simulink model "bh_test_J_DBL_pend"  (R2016b)
settings: Solver=ode15s  StartTime=0.0  StopTime=30  MaxStep=0.01  RelTol=1e-5  EnableMultiTasking=on
undefined symbols (not defined in the file or in its folder): g, L1x, L1y, L1z, L2x, L2y, L2z, mass1, mass2, theta1_0, theta2_0, X, Y, Z
undefined symbols (not defined in the file): dt
libraries: nesl_utility x14, sm_lib x12, simulink_extras x4, simulink x2
settings Model: Creator=bhorton  LastModifiedBy=bhorton
settings OptimizationCC: LifeSpan=inf
settings DebuggingCC: SFUnexpectedBacktrackingDiag=warning  SFNoUnconditionalDefaultTransitionDiag=warning  SFExecutionAtInitializationDiag=none
settings GRTTargetCC: TargetLangStandard=C89/C90 (ANSI)  GeneratePreprocessorConditionals=Disable all
settings ConfigComp: CovMetricSettings=dw  CovHtmlReporting=on  CovSaveCumulativeToWorkspaceVar=on  CovSaveSingleToWorkspaceVar=on  CovExternalEMLEnable=off

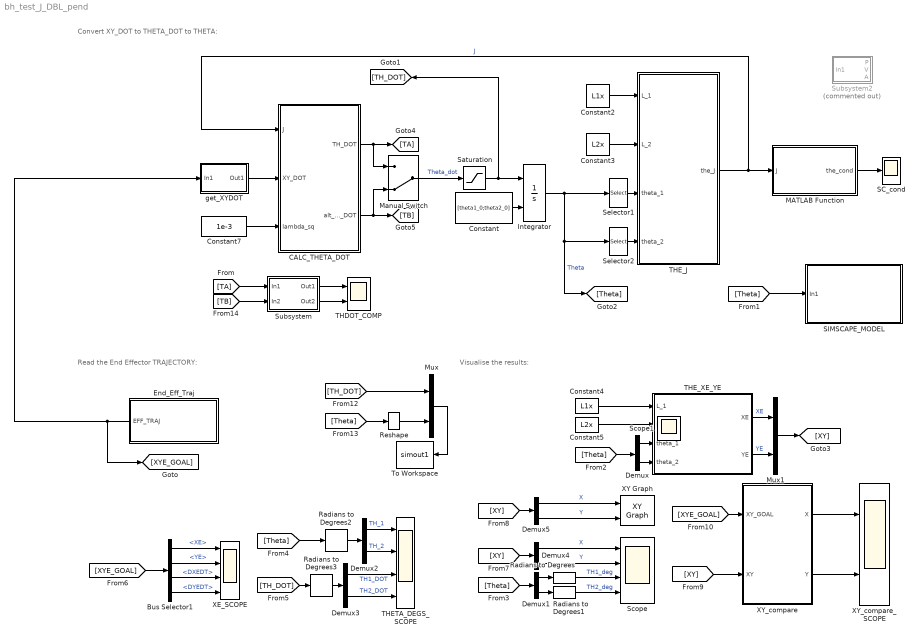
== system bh_test_J_DBL_pend ==
  note: Visualise the results:
  note: Read the End Effector TRAJECTORY:
  note: Convert XY_DOT to THETA_DOT to THETA:
  Bus Selector1 : BusSelector  OutputSignals=XE,YE,DXEDT,DYEDT
  CALC_THETA_DOT : MATLAB Function  TreatAsAtomicUnit=on
  Constant : Constant  Value=[theta1_0;theta2_0]  VectorParams1D=off
  Constant2 : Constant  Value=L1x
  Constant3 : Constant  Value=L2x
  Constant4 : Constant  Value=L1x
  Constant5 : Constant  Value=L2x
  Constant7 : Constant  Value=1e-3
  Demux{,1..5} (6 alike) : Demux  Outputs=2
  End_Eff_Traj : Subsystem
  Integrator : Integrator  InitialConditionSource=external
  MATLAB Function : MATLAB Function  TreatAsAtomicUnit=on
  Manual Switch : ManualSwitch  CurrentSetting=0
  Mux : Mux  Inputs=2
  Mux1 : Mux  Inputs=2
  Radians to Degrees{,1..3} (4 alike) : simulink_extras/Transformations/Radians to Degrees
  Reshape : Reshape
  SC_cond : Scope
  SIMSCAPE_MODEL : Subsystem
  Saturation : Saturate  UpperLimit=6  LowerLimit=-6
  Scope : Scope  NumInputPorts=4
  Selector1 : Selector  InputPortWidth=2  IndexOptions=Index vector (dialog)  Indices=1  OutputSizes=1
  Selector2 : Selector  InputPortWidth=2  IndexOptions=Index vector (dialog)  Indices=2  OutputSizes=1
  Subsystem : Subsystem
  Subsystem2 : Subsystem  Commented=on
  THDOT_COMP : Scope  NumInputPorts=2
  THETA_DEGS_SCOPE : Scope  NumInputPorts=4
  THE_J : MATLAB Function  TreatAsAtomicUnit=on
  THE_XE_YE : MATLAB Function  TreatAsAtomicUnit=on
  To Workspace : ToWorkspace  VariableName=simout1  SaveFormat=Structure With Time  SampleTime=-1
      settings: Save2DSignal=2-D array (concatenate along first dimension)
  XE_SCOPE : Scope  NumInputPorts=4
  XY Graph : simulink/Sinks/XY Graph  xmin=0  xmax=1.6  ymin=0  ymax=1.6  st=-1
  XY_compare : Subsystem
  XY_compare_SCOPE : Scope  NumInputPorts=2
  get_XYDOT : Subsystem
  Scope1 : Scope
  wires:
  Constant/1 -> Integrator/2
  Constant3/1 -> THE_J/2(L_2)
  Constant2/1 -> THE_J/1(L_1)
  THE_J/1(the_J) -> CALC_THETA_DOT/1(J), MATLAB Function/1(J)  "J"
  get_XYDOT/1(Out1) -> CALC_THETA_DOT/2(XY_DOT)
  Manual Switch/1 -> Saturation/1  "Theta_dot"
  Constant5/1 -> THE_XE_YE/2(L_2)
  Constant4/1 -> THE_XE_YE/1(L_1)
  MATLAB Function/1(the_cond) -> SC_cond/1
  Integrator/1 -> Selector2/1, [Theta], Selector1/1  "Theta"
  Selector1/1 -> THE_J/3(theta_1)
  Selector2/1 -> THE_J/4(theta_2)
  Demux/1 -> THE_XE_YE/3(theta_1)
  Demux/2 -> THE_XE_YE/4(theta_2)
  [Theta] -> Demux/1
  [Theta] -> Demux1/1
  Demux1/1 -> Radians to Degrees/1
  Demux1/2 -> Radians to Degrees1/1
  [Theta] -> SIMSCAPE_MODEL/1(In1)
  Demux2/1 -> THETA_DEGS_SCOPE/1  "TH_1"
  Demux2/2 -> THETA_DEGS_SCOPE/2  "TH_2"
  [Theta] -> Radians to Degrees2/1
  Demux3/1 -> THETA_DEGS_SCOPE/3  "TH1_DOT"
  Demux3/2 -> THETA_DEGS_SCOPE/4  "TH2_DOT"
  [TH_DOT] -> Radians to Degrees3/1
  Radians to Degrees2/1 -> Demux2/1
  Radians to Degrees3/1 -> Demux3/1
  [XYE_GOAL] -> Bus Selector1/1
  Bus Selector1/1 -> XE_SCOPE/1  "<XE>"
  Bus Selector1/2 -> XE_SCOPE/2  "<YE>"
  Bus Selector1/3 -> XE_SCOPE/3  "<DXEDT>"
  Bus Selector1/4 -> XE_SCOPE/4  "<DYEDT>"
  THE_XE_YE/1(XE) -> Mux1/1  "XE"
  THE_XE_YE/2(YE) -> Mux1/2  "YE"
  Mux1/1 -> [XY]
  Radians to Degrees1/1 -> Scope/4  "TH2_deg"
  Radians to Degrees/1 -> Scope/3  "TH1_deg"
  [XY] -> Demux4/1
  Demux4/1 -> Scope/1  "X"
  Demux4/2 -> Scope/2  "Y"
  [XY] -> Demux5/1
  Demux5/1 -> XY Graph/1  "X"
  Demux5/2 -> XY Graph/2  "Y"
  [XY] -> XY_compare/2(XY)
  [XYE_GOAL] -> XY_compare/1(XY_GOAL)
  XY_compare/2(Y) -> XY_compare_SCOPE/2
  XY_compare/1(X) -> XY_compare_SCOPE/1
  End_Eff_Traj/1(EFF_TRAJ) -> [XYE_GOAL], get_XYDOT/1(In1)
  Saturation/1 -> [TH_DOT], Integrator/1
  [TH_DOT] -> Mux/1
  Mux/1 -> To Workspace/1
  [Theta] -> Reshape/1
  Reshape/1 -> Mux/2
  [TB] -> Subsystem/2(In2)
  [TA] -> Subsystem/1(In1)
  Subsystem/1(Out1) -> THDOT_COMP/1
  Subsystem/2(Out2) -> THDOT_COMP/2
  CALC_THETA_DOT/1(TH_DOT) -> [TA], Manual Switch/1
  CALC_THETA_DOT/2(alt_TH_DOT) -> [TB], Manual Switch/2
  Constant7/1 -> CALC_THETA_DOT/3(lambda_sq)

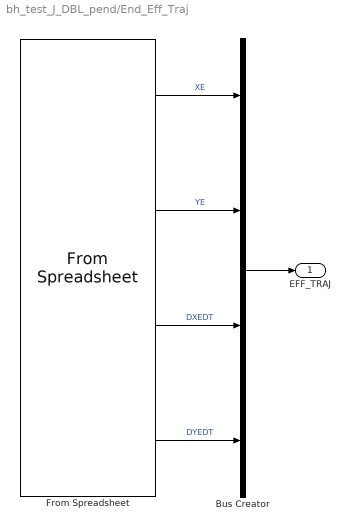
== system bh_test_J_DBL_pend/End_Eff_Traj ==
  Bus Creator : BusCreator  Inputs=4
  From Spreadsheet : FromSpreadsheet  FileName=bh_hello_complete.xlsx  SheetName=COMP_SPLINE  SampleTime=-1  ExtrapolationBeforeFirstDataPoint=Hold first value  ExtrapolationAfterLastDataPoint=Hold last value
  EFF_TRAJ : Outport
  wires:
  From Spreadsheet/2 -> Bus Creator/2  "YE"
  From Spreadsheet/3 -> Bus Creator/3  "DXEDT"
  From Spreadsheet/1 -> Bus Creator/1  "XE"
  From Spreadsheet/4 -> Bus Creator/4  "DYEDT"
  Bus Creator/1 -> EFF_TRAJ/1

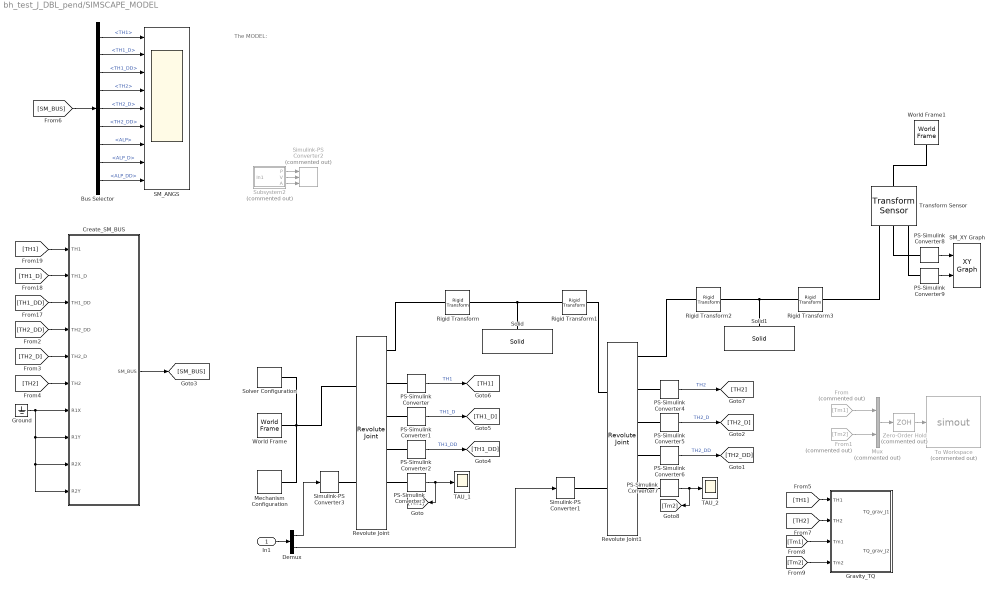
== system bh_test_J_DBL_pend/SIMSCAPE_MODEL ==
  note: The MODEL:
  In1 : Inport
  Bus Selector : BusSelector  OutputSignals=TH1,TH1_D,TH1_DD,TH2,TH2_D,TH2_DD,ALP,ALP_D,ALP_DD
  Create_SM_BUS : Subsystem
  Demux : Demux  Outputs=2
  From : From  Commented=on  GotoTag=Tm1
  From1 : From  Commented=on  GotoTag=Tm2
  Gravity_TQ : Subsystem
  Ground : Ground
  Mechanism Configuration : sm_lib/Utilities/Mechanism Configuration  UniformGravity=Constant  GravityVector=[0 -9.80665 0 ]  GravityUnits=m/s^2  LinearizationDelta=0.001
  Mux : Mux  Commented=on  Inputs=2
  PS-Simulink Converter : nesl_utility/PS-Simulink Converter  PhysicalDomain=network_engine_domain  SubClassName=ps_output  LeftPortType=input  RightPortType=output  PseudoPeriodic=off  Frequencies=[]  Unit=rad  AffineConversion=off
  PS-Simulink Converter1 : nesl_utility/PS-Simulink Converter  PhysicalDomain=network_engine_domain  SubClassName=ps_output  LeftPortType=input  RightPortType=output  PseudoPeriodic=off  Frequencies=[]  Unit=rad/s  AffineConversion=off
  PS-Simulink Converter2 : nesl_utility/PS-Simulink Converter  PhysicalDomain=network_engine_domain  SubClassName=ps_output  LeftPortType=input  RightPortType=output  PseudoPeriodic=off  Frequencies=[]  Unit=rad/s^2  AffineConversion=off
  PS-Simulink Converter3 : nesl_utility/PS-Simulink Converter  PhysicalDomain=network_engine_domain  SubClassName=ps_output  LeftPortType=input  RightPortType=output  PseudoPeriodic=off  Frequencies=[]  Unit=N*m  AffineConversion=off
  PS-Simulink Converter4 : nesl_utility/PS-Simulink Converter  PhysicalDomain=network_engine_domain  SubClassName=ps_output  LeftPortType=input  RightPortType=output  PseudoPeriodic=off  Frequencies=[]  Unit=rad  AffineConversion=off
  PS-Simulink Converter5 : nesl_utility/PS-Simulink Converter  PhysicalDomain=network_engine_domain  SubClassName=ps_output  LeftPortType=input  RightPortType=output  PseudoPeriodic=off  Frequencies=[]  Unit=rad/s  AffineConversion=off
  PS-Simulink Converter6 : nesl_utility/PS-Simulink Converter  PhysicalDomain=network_engine_domain  SubClassName=ps_output  LeftPortType=input  RightPortType=output  PseudoPeriodic=off  Frequencies=[]  Unit=rad/s^2  AffineConversion=off
  PS-Simulink Converter7 : nesl_utility/PS-Simulink Converter  PhysicalDomain=network_engine_domain  SubClassName=ps_output  LeftPortType=input  RightPortType=output  PseudoPeriodic=off  Frequencies=[]  Unit=N*m  AffineConversion=off
  PS-Simulink Converter8 : nesl_utility/PS-Simulink Converter  PhysicalDomain=network_engine_domain  SubClassName=ps_output  LeftPortType=input  RightPortType=output  PseudoPeriodic=off  Frequencies=[]  Unit=m  AffineConversion=off
  PS-Simulink Converter9 : nesl_utility/PS-Simulink Converter  PhysicalDomain=network_engine_domain  SubClassName=ps_output  LeftPortType=input  RightPortType=output  PseudoPeriodic=off  Frequencies=[]  Unit=m  AffineConversion=off
  Revolute Joint : sm_lib/Joints/Revolute Joint  SenseConstraintForce=on  SenseConstraintForceX=off  SenseConstraintForceY=off  SenseConstraintForceZ=off  SenseConstraintTorque=off  SenseConstraintTorqueX=off  SenseConstraintTorqueY=off  SenseConstraintTorqueZ=off  SenseTotalForce=off  SenseTotalForceX=off  SenseTotalForceY=off  SenseTotalForceZ=off  SenseTotalTorque=off  SenseTotalTorqueX=off  SenseTotalTorqueY=off  SenseTotalTorqueZ=off  CompositeWrenchDir=BaseOnFollower  CompositeWrenchFrame=BaseFrame  EquilibriumPosition=0  EquilibriumPositionUnits=deg  SpringStiffness=0  SpringStiffnessUnits=N*m/deg  DampingCoefficient=b1_damp  DampingCoefficientUnits=N*m/(rad/s)  TorqueActuationMode=ComputedTorque  MotionActuationMode=InputMotion  SensePosition=on  SenseVelocity=on  SenseAcceleration=on  SenseTorqueForce=on  PositionTargetSpecify=off  PositionTargetPriority=Low  PositionTargetValue=0  PositionTargetValueUnits=rad  VelocityTargetSpecify=off  VelocityTargetPriority=High  VelocityTargetValue=0  VelocityTargetValueUnits=rad/s
  Revolute Joint1 : sm_lib/Joints/Revolute Joint  SenseConstraintForce=on  SenseConstraintForceX=off  SenseConstraintForceY=off  SenseConstraintForceZ=off  SenseConstraintTorque=off  SenseConstraintTorqueX=off  SenseConstraintTorqueY=off  SenseConstraintTorqueZ=off  SenseTotalForce=off  SenseTotalForceX=off  SenseTotalForceY=off  SenseTotalForceZ=off  SenseTotalTorque=off  SenseTotalTorqueX=off  SenseTotalTorqueY=off  SenseTotalTorqueZ=off  CompositeWrenchDir=BaseOnFollower  CompositeWrenchFrame=FollowerFrame  EquilibriumPosition=0  EquilibriumPositionUnits=deg  SpringStiffness=0  SpringStiffnessUnits=N*m/deg  DampingCoefficient=b2_damp  DampingCoefficientUnits=N*m/(rad/s)  TorqueActuationMode=ComputedTorque  MotionActuationMode=InputMotion  SensePosition=on  SenseVelocity=on  SenseAcceleration=on  SenseTorqueForce=on  PositionTargetSpecify=off  PositionTargetPriority=Low  PositionTargetValue=0  PositionTargetValueUnits=rad  VelocityTargetSpecify=off  VelocityTargetPriority=High  VelocityTargetValue=0  VelocityTargetValueUnits=rad/s
  Rigid Transform : sm_lib/Frames and Transforms/Rigid Transform  TranslationMethod=StandardAxis  TranslationStandardOffset=L1x/2  TranslationLengthUnit=m  TranslationStandardAxis=+X  TranslationCartesianOffset=[0 0 0]  TranslationROffset=0  TranslationROffsetUnits=m  TranslationZOffset=0  TranslationZOffsetUnits=m  TranslationThetaOffset=0  TranslationThetaOffsetUnits=deg  RotationMethod=None  RotationAngleUnits=deg  RotationStandardAxis=+Z  RotationAngle=0.0  RotationArbitraryAxis=[0 0 1]  FollAlignAxisA=+X  BaseAlignAxisA=+Y  FollAlignAxisB=+Y  BaseAlignAxisB=+Z  RotationSequenceAxes=FollowerAxes  RotationSequence=XYX  RotationSequenceAngles=[0 0 0]  RotationSequenceAnglesUnits=deg  RotationMatrix=[1 0 0; 0 1 0; 0 0 1]
  Rigid Transform1 : sm_lib/Frames and Transforms/Rigid Transform  TranslationMethod=StandardAxis  TranslationStandardOffset=L1x/2  TranslationLengthUnit=m  TranslationStandardAxis=+X  TranslationCartesianOffset=[0 0 0]  TranslationROffset=0  TranslationROffsetUnits=m  TranslationZOffset=0  TranslationZOffsetUnits=m  TranslationThetaOffset=0  TranslationThetaOffsetUnits=deg  RotationMethod=None  RotationAngleUnits=deg  RotationStandardAxis=+Z  RotationAngle=0.0  RotationArbitraryAxis=[0 0 1]  FollAlignAxisA=+X  BaseAlignAxisA=+Y  FollAlignAxisB=+Y  BaseAlignAxisB=+Z  RotationSequenceAxes=FollowerAxes  RotationSequence=XYX  RotationSequenceAngles=[0 0 0]  RotationSequenceAnglesUnits=deg  RotationMatrix=[1 0 0; 0 1 0; 0 0 1]
  Rigid Transform2 : sm_lib/Frames and Transforms/Rigid Transform  TranslationMethod=StandardAxis  TranslationStandardOffset=L2x/2  TranslationLengthUnit=m  TranslationStandardAxis=+X  TranslationCartesianOffset=[0 0 0]  TranslationROffset=0  TranslationROffsetUnits=m  TranslationZOffset=0  TranslationZOffsetUnits=m  TranslationThetaOffset=0  TranslationThetaOffsetUnits=deg  RotationMethod=None  RotationAngleUnits=deg  RotationStandardAxis=+Z  RotationAngle=0.0  RotationArbitraryAxis=[0 0 1]  FollAlignAxisA=+X  BaseAlignAxisA=+Y  FollAlignAxisB=+Y  BaseAlignAxisB=+Z  RotationSequenceAxes=FollowerAxes  RotationSequence=XYX  RotationSequenceAngles=[0 0 0]  RotationSequenceAnglesUnits=deg  RotationMatrix=[1 0 0; 0 1 0; 0 0 1]
  Rigid Transform3 : sm_lib/Frames and Transforms/Rigid Transform  TranslationMethod=StandardAxis  TranslationStandardOffset=L2x/2  TranslationLengthUnit=m  TranslationStandardAxis=+X  TranslationCartesianOffset=[0 0 0]  TranslationROffset=0  TranslationROffsetUnits=m  TranslationZOffset=0  TranslationZOffsetUnits=m  TranslationThetaOffset=0  TranslationThetaOffsetUnits=deg  RotationMethod=None  RotationAngleUnits=deg  RotationStandardAxis=+Z  RotationAngle=0.0  RotationArbitraryAxis=[0 0 1]  FollAlignAxisA=+X  BaseAlignAxisA=+Y  FollAlignAxisB=+Y  BaseAlignAxisB=+Z  RotationSequenceAxes=FollowerAxes  RotationSequence=XYX  RotationSequenceAngles=[0 0 0]  RotationSequenceAnglesUnits=deg  RotationMatrix=[1 0 0; 0 1 0; 0 0 1]
  SM_ANGS : Scope  NumInputPorts=9
  SM_XY Graph : simulink/Sinks/XY Graph  xmin=0  xmax=1.6  ymin=0  ymax=1.6  st=-1
  Simulink-PS Converter1 : nesl_utility/Simulink-PS Converter  PhysicalDomain=network_engine_domain  SubClassName=ps_input  LeftPortType=input  RightPortType=output  PseudoPeriodic=off  Frequencies=[]  NoiseDistribution=none  NoiseParameters=[]  Unit=rad  AffineConversion=off  InputFiltering=on  SimscapeFilterOrder=2  InputFilterTimeConstant=0.05  UdotUserProvided=2
  Simulink-PS Converter2 : nesl_utility/Simulink-PS Converter  Commented=on  PhysicalDomain=network_engine_domain  SubClassName=ps_input  LeftPortType=input  RightPortType=output  PseudoPeriodic=off  Frequencies=[]  NoiseDistribution=none  NoiseParameters=[]  Unit=rad  AffineConversion=off  InputFiltering=derivs  SimscapeFilterOrder=2  InputFilterTimeConstant=0.01  UdotUserProvided=2
  Simulink-PS Converter3 : nesl_utility/Simulink-PS Converter  PhysicalDomain=network_engine_domain  SubClassName=ps_input  LeftPortType=input  RightPortType=output  PseudoPeriodic=off  Frequencies=[]  NoiseDistribution=none  NoiseParameters=[]  Unit=rad  AffineConversion=off  InputFiltering=on  SimscapeFilterOrder=2  InputFilterTimeConstant=0.05  UdotUserProvided=2
  Solid : sm_lib/Body Elements/Solid  InertiaType=CalculateFromGeometry  Mass=1  MassUnits=kg  CenterOfMass=[0 0 0]  CenterOfMassUnits=m  MomentsOfInertia=[1 1 1]  MomentsOfInertiaUnits=kg*m^2  ProductsOfInertia=[0 0 0]  ProductsOfInertiaUnits=kg*m^2  DensityBased=on  Density=density  DensityUnits=kg/(m^3)  DoExposeReferenceFrame=on  SerializedFrames=<Frames/>  GraphicType=FromGeometry  MarkerShape=Sphere  MarkerSize=10  GraphicVisPropType=SimpleVisualProperties  GraphicDiffuseColor=[0.8 0.8 1.0]  GraphicSpecularColor=[0.5 0.5 0.5 1.0]  GraphicAmbientColor=[0.15 0.15 0.15 1.0]  GraphicEmissiveColor=[0.0 0.0 0.0 1.0]  GraphicShininess=75  GraphicOpacity=1.0  GeometryShape=Brick  RectangleSize=[1 1]  RectangleSizeUnits=m  BrickDimensions=[L1x, L1y, L1z ]  BrickDimensionUnits=m  CylinderRadius=1  CylinderRadiusUnits=m  CylinderLength=1  CylinderLengthUnits=m  SphereRadius=1  SphereRadiusUnits=m  EllipsoidRadii=[1 1 1]  EllipsoidRadiiUnits=m  ExtrusionCrossSection=[1 1; -1 1; -1 -1; 1 -1]  ExtrusionCrossSectionUnits=m  ExtrusionLength=1  ExtrusionLengthUnits=m  PolygonNumSides=3  PolygonOuterRadius=1  PolygonOuterRadiusUnits=m  ExtGeomFileType=STEP  ExtGeomFileUnits=m  RevolutionCrossSection=[1 1; 1 -1; 2 -1; 2 1]  RevolutionCrossSectionUnits=m  RevolutionExtent=Full  RevolutionAngle=180  RevolutionAngleUnits=deg
  Solid1 : sm_lib/Body Elements/Solid  InertiaType=CalculateFromGeometry  Mass=1  MassUnits=kg  CenterOfMass=[0 0 0]  CenterOfMassUnits=m  MomentsOfInertia=[1 1 1]  MomentsOfInertiaUnits=kg*m^2  ProductsOfInertia=[0 0 0]  ProductsOfInertiaUnits=kg*m^2  DensityBased=on  Density=density  DensityUnits=kg/(m^3)  DoExposeReferenceFrame=on  SerializedFrames=<Frames/>  GraphicType=FromGeometry  MarkerShape=Sphere  MarkerSize=10  GraphicVisPropType=SimpleVisualProperties  GraphicDiffuseColor=[1.0 0.6 1.0]  GraphicSpecularColor=[0.5 0.5 0.5 1.0]  GraphicAmbientColor=[0.15 0.15 0.15 1.0]  GraphicEmissiveColor=[0.0 0.0 0.0 1.0]  GraphicShininess=75  GraphicOpacity=1.0  GeometryShape=Brick  RectangleSize=[1 1]  RectangleSizeUnits=m  BrickDimensions=[L2x, L2y, L2z ]  BrickDimensionUnits=m  CylinderRadius=1  CylinderRadiusUnits=m  CylinderLength=1  CylinderLengthUnits=m  SphereRadius=1  SphereRadiusUnits=m  EllipsoidRadii=[1 1 1]  EllipsoidRadiiUnits=m  ExtrusionCrossSection=[1 1; -1 1; -1 -1; 1 -1]  ExtrusionCrossSectionUnits=m  ExtrusionLength=1  ExtrusionLengthUnits=m  PolygonNumSides=3  PolygonOuterRadius=1  PolygonOuterRadiusUnits=m  ExtGeomFileType=STEP  ExtGeomFileUnits=m  RevolutionCrossSection=[1 1; 1 -1; 2 -1; 2 1]  RevolutionCrossSectionUnits=m  RevolutionExtent=Full  RevolutionAngle=180  RevolutionAngleUnits=deg
  Solver Configuration : nesl_utility/Solver Configuration  PhysicalDomain=network_engine_domain  SubClassName=solver  LeftPortType=input  RightPortType=generic  Accelerate=off  Tones=[]  Harmonics=[]  SimulateNoise=off  Profile=off  UseLocalSampling=off  EnableSwitchedLinearOptims=on  FrequencyDomain=off  UseCCode=off  RelTol=0.001  AbsTol=1e-06  MinStep=1e-09  ToWorkspace=off  RevertToSquareIcSolve=off  NumHomotopyIterations=100  PhasorMode=off  PhasorModeNumHarmonics=1  OverrideAbsTol=off  DoDC=off  ResidualTolerance=1e-09  UseLocalSolver=off  LocalSolverChoice=NE_BACKWARD_EULER_ADVANCER  LocalSolverSampleTime=0.001  DoFixedCost=off  MaxNonlinIter=3  MaxModeIter=2  LinearAlgebra=Sparse  DelaysMemoryBudget=1024  AutomaticFiltering=on  FilteringTimeConstant=0.001
  Subsystem2 : Subsystem  Commented=on
  TAU_1 : Scope
  TAU_2 : Scope
  To Workspace : ToWorkspace  Commented=on  VariableName=simout  SaveFormat=Structure With Time  SampleTime=-1
  Transform Sensor : sm_lib/Frames and Transforms/Transform Sensor  MeasurementFrame=World  SenseAngle=off  SenseAxis=off  SenseAngle1=off  SenseAngle2=off  SenseAngle3=off  SenseQ=off  SenseR=off  SenseOmegaX=off  SenseOmegaY=off  SenseOmegaZ=off  SenseOmega1=off  SenseOmega2=off  SenseOmega3=off  SenseQDot=off  SenseRDot=off  SenseAlphaX=off  SenseAlphaY=off  SenseAlphaZ=off  SenseAlpha1=off  SenseAlpha2=off  SenseAlpha3=off  SenseQDDot=off  SenseRDDot=off  SenseX=on  SenseY=on  SenseZ=off  SenseRad=off  SenseAzim=off  SenseDist=off  SenseInc=off  SenseXDot=off  SenseYDot=off  SenseZDot=off  SenseRadDot=off  SenseAzimDot=off  SenseDistDot=off  SenseIncDot=off  SenseXDDot=off  SenseYDDot=off  SenseZDDot=off  SenseRadDDot=off  SenseAzimDDot=off  SenseDistDDot=off  SenseIncDDot=off
  World Frame : sm_lib/Frames and Transforms/World Frame
  World Frame1 : sm_lib/Frames and Transforms/World Frame
  Zero-Order Hold : ZeroOrderHold  Commented=on  SampleTime=0.01
  wires:
  PS-Simulink Converter/1 -> [TH1]  "TH1"
  PS-Simulink Converter2/1 -> [TH1_DD]  "TH1_DD"
  PS-Simulink Converter1/1 -> [TH1_D]  "TH1_D"
  PS-Simulink Converter4/1 -> [TH2]  "TH2"
  PS-Simulink Converter6/1 -> [TH2_DD]  "TH2_DD"
  PS-Simulink Converter5/1 -> [TH2_D]  "TH2_D"
  [TH2_D] -> Create_SM_BUS/5(TH2_D)
  [TH1_D] -> Create_SM_BUS/2(TH1_D)
  [TH2_DD] -> Create_SM_BUS/4(TH2_DD)
  [TH2] -> Create_SM_BUS/6(TH2)
  [TH1_DD] -> Create_SM_BUS/3(TH1_DD)
  [TH1] -> Create_SM_BUS/1(TH1)
  Create_SM_BUS/1(SM_BUS) -> [SM_BUS]
  [SM_BUS] -> Bus Selector/1
  Bus Selector/2 -> SM_ANGS/2  "<TH1_D>"
  Bus Selector/3 -> SM_ANGS/3  "<TH1_DD>"
  Bus Selector/1 -> SM_ANGS/1  "<TH1>"
  Bus Selector/4 -> SM_ANGS/4  "<TH2>"
  Bus Selector/5 -> SM_ANGS/5  "<TH2_D>"
  Bus Selector/6 -> SM_ANGS/6  "<TH2_DD>"
  Bus Selector/7 -> SM_ANGS/7  "<ALP>"
  Bus Selector/8 -> SM_ANGS/8  "<ALP_D>"
  Bus Selector/9 -> SM_ANGS/9  "<ALP_DD>"
  Ground/1 -> Create_SM_BUS/8(R1Y), Create_SM_BUS/9(R2X), Create_SM_BUS/10(R2Y), Create_SM_BUS/7(R1X)
  In1/1 -> Demux/1
  PS-Simulink Converter7/1 -> [Tm2], TAU_2/1
  PS-Simulink Converter3/1 -> [Tm1], TAU_1/1
  Demux/1 -> Simulink-PS Converter3/1
  Demux/2 -> Simulink-PS Converter1/1
  Subsystem2/1(P) -> Simulink-PS Converter2/1
  Subsystem2/2(V) -> Simulink-PS Converter2/2
  Subsystem2/3(A) -> Simulink-PS Converter2/3
  PS-Simulink Converter8/1 -> SM_XY Graph/1
  PS-Simulink Converter9/1 -> SM_XY Graph/2
  Mux/1 -> Zero-Order Hold/1
  From/1 -> Mux/1
  From1/1 -> Mux/2
  Zero-Order Hold/1 -> To Workspace/1
  [TH1] -> Gravity_TQ/1(TH1)
  [TH2] -> Gravity_TQ/2(TH2)
  [Tm2] -> Gravity_TQ/4(Tm2)
  [Tm1] -> Gravity_TQ/3(Tm1)
  connections:
  World Frame/RConn1 -- Revolute Joint/LConn1 -- Solver Configuration/RConn1 -- Mechanism Configuration/RConn1
  Solid/RConn1 -- Rigid Transform1/LConn1 -- Rigid Transform/RConn1
  Revolute Joint/RConn3 -- PS-Simulink Converter1/LConn1
  Revolute Joint/RConn4 -- PS-Simulink Converter2/LConn1
  Rigid Transform/LConn1 -- Revolute Joint/RConn1
  PS-Simulink Converter/LConn1 -- Revolute Joint/RConn2
  Revolute Joint1/LConn1 -- Rigid Transform1/RConn1
  Revolute Joint1/RConn3 -- PS-Simulink Converter5/LConn1
  Revolute Joint1/RConn2 -- PS-Simulink Converter4/LConn1
  Revolute Joint1/RConn4 -- PS-Simulink Converter6/LConn1
  Rigid Transform2/RConn1 -- Rigid Transform3/LConn1 -- Solid1/RConn1
  Rigid Transform2/LConn1 -- Revolute Joint1/RConn1
  Simulink-PS Converter3/RConn1 -- Revolute Joint/LConn2
  Simulink-PS Converter1/RConn1 -- Revolute Joint1/LConn2
  PS-Simulink Converter3/LConn1 -- Revolute Joint/RConn5
  Revolute Joint1/RConn5 -- PS-Simulink Converter7/LConn1
  World Frame1/RConn1 -- Transform Sensor/LConn1
  Transform Sensor/RConn1 -- Rigid Transform3/RConn1
  PS-Simulink Converter8/LConn1 -- Transform Sensor/RConn2
  PS-Simulink Converter9/LConn1 -- Transform Sensor/RConn3

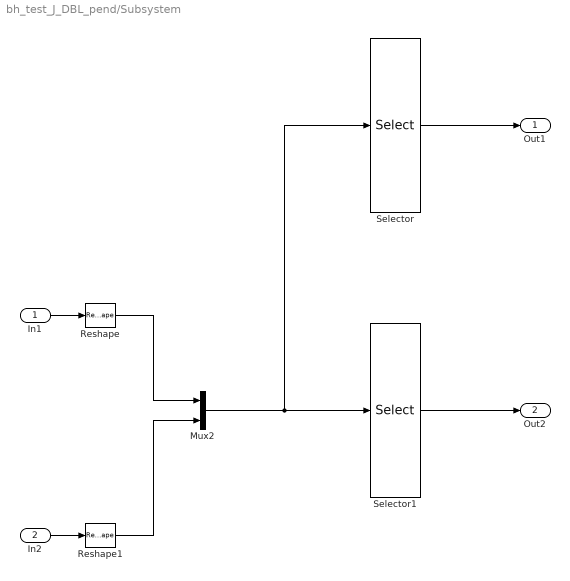
== system bh_test_J_DBL_pend/Subsystem ==
  In1 : Inport
  In2 : Inport  Port=2
  Mux2 : Mux  Inputs=2
  Reshape : Reshape  OutputDimensionality=Column vector (2-D)
  Reshape1 : Reshape  OutputDimensionality=Column vector (2-D)
  Selector : Selector  InputPortWidth=4  IndexOptions=Index vector (dialog)  Indices=[1 3]  OutputSizes=1
  Selector1 : Selector  InputPortWidth=4  IndexOptions=Index vector (dialog)  Indices=[2 4]  OutputSizes=1
  Out1 : Outport
  Out2 : Outport  Port=2
  wires:
  In1/1 -> Reshape/1
  In2/1 -> Reshape1/1
  Reshape/1 -> Mux2/1
  Reshape1/1 -> Mux2/2
  Selector1/1 -> Out2/1
  Selector/1 -> Out1/1
  Mux2/1 -> Selector/1, Selector1/1

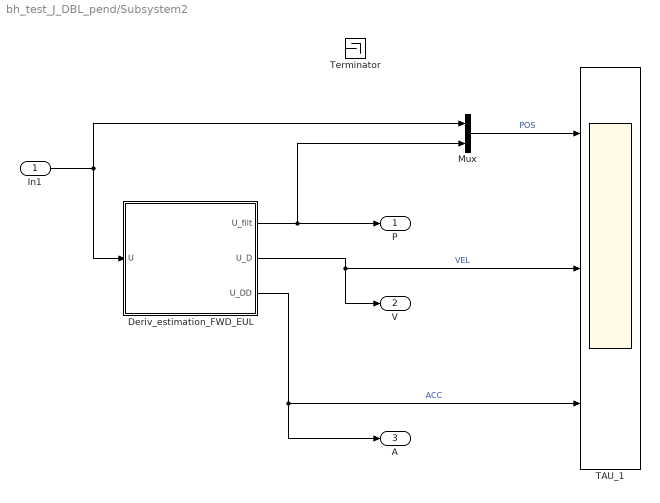
== system bh_test_J_DBL_pend/Subsystem2 ==
  In1 : Inport
  Deriv_estimation_FWD_EUL : Subsystem  mask(Derivative Estimation){wn=2*pi*10, p=1, dt=dt}
      mask prompts: wn "Natural frequency, wn (rad/sec)"; p "Damping ratio, p"; dt "Sample time, dt (secs)"
      mask help: A simple derivative estimator using a 2nd order representation between input and output.
      mask init:
      | str1 = sprintf('wn = %.2f', wn);
      | str2 = sprintf('p  = %.2f', p);
      | str3 = sprintf('dt = %.2f', dt);
      | str = char(str1,str2,str3);
      mask Display: disp(str)
  Mux : Mux  Inputs=2
  TAU_1 : Scope  NumInputPorts=3
  Terminator : Terminator
  P : Outport
  V : Outport  Port=2
  A : Outport  Port=3
  wires:
  In1/1 -> Deriv_estimation_FWD_EUL/1(U), Mux/1
  Deriv_estimation_FWD_EUL/1(U_filt) -> Mux/2, P/1
  Deriv_estimation_FWD_EUL/2(U_D) -> TAU_1/2, V/1  "VEL"
  Deriv_estimation_FWD_EUL/3(U_DD) -> TAU_1/3, A/1  "ACC"
  Mux/1 -> TAU_1/1  "POS"

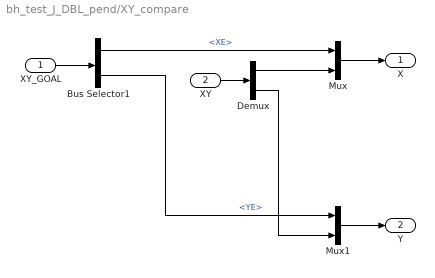
== system bh_test_J_DBL_pend/XY_compare ==
  XY_GOAL : Inport
  XY : Inport  Port=2
  Bus Selector1 : BusSelector  OutputSignals=XE,YE
  Demux : Demux  Outputs=2
  Mux : Mux  Inputs=2
  Mux1 : Mux  Inputs=2
  X : Outport
  Y : Outport  Port=2
  wires:
  XY_GOAL/1 -> Bus Selector1/1
  XY/1 -> Demux/1
  Bus Selector1/1 -> Mux/1  "<XE>"
  Demux/1 -> Mux/2
  Bus Selector1/2 -> Mux1/1  "<YE>"
  Demux/2 -> Mux1/2
  Mux/1 -> X/1
  Mux1/1 -> Y/1

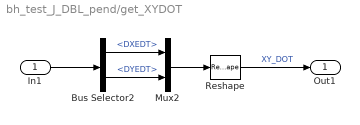
== system bh_test_J_DBL_pend/get_XYDOT ==
  In1 : Inport
  Bus Selector2 : BusSelector  OutputSignals=DXEDT,DYEDT
  Mux2 : Mux  Inputs=2
  Reshape : Reshape  OutputDimensionality=Column vector (2-D)
  Out1 : Outport
  wires:
  Bus Selector2/1 -> Mux2/1  "<DXEDT>"
  Bus Selector2/2 -> Mux2/2  "<DYEDT>"
  In1/1 -> Bus Selector2/1
  Mux2/1 -> Reshape/1
  Reshape/1 -> Out1/1  "XY_DOT"

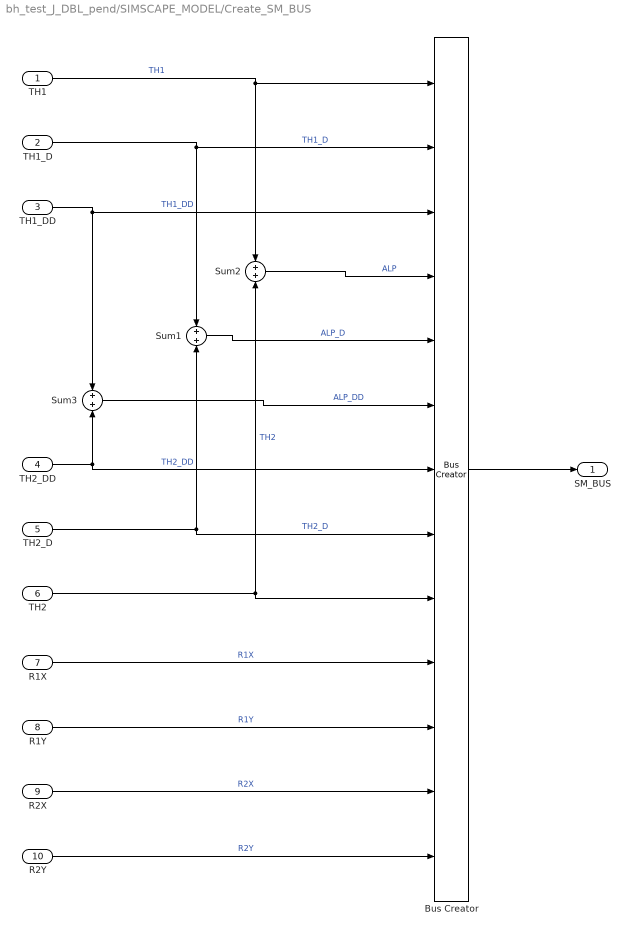
== system bh_test_J_DBL_pend/SIMSCAPE_MODEL/Create_SM_BUS ==
  TH1 : Inport
  TH1_D : Inport  Port=2
  TH1_DD : Inport  Port=3
  TH2_DD : Inport  Port=4
  TH2_D : Inport  Port=5
  TH2 : Inport  Port=6
  R1X : Inport  Port=7
  R1Y : Inport  Port=8
  R2X : Inport  Port=9
  R2Y : Inport  Port=10
  Bus Creator : BusCreator  Inputs=13
  Sum1 : Sum  Inputs=+|+
  Sum2 : Sum  Inputs=+|+
  Sum3 : Sum  Inputs=+|+
  SM_BUS : Outport
  wires:
  TH2_DD/1 -> Bus Creator/7, Sum3/2  "TH2_DD"
  TH1_DD/1 -> Sum3/1, Bus Creator/3  "TH1_DD"
  TH1_D/1 -> Bus Creator/2, Sum1/1  "TH1_D"
  TH2_D/1 -> Bus Creator/8, Sum1/2  "TH2_D"
  TH1/1 -> Bus Creator/1, Sum2/1  "TH1"
  TH2/1 -> Bus Creator/9, Sum2/2  "TH2"
  Sum2/1 -> Bus Creator/4  "ALP"
  Sum1/1 -> Bus Creator/5  "ALP_D"
  Sum3/1 -> Bus Creator/6  "ALP_DD"
  Bus Creator/1 -> SM_BUS/1
  R1Y/1 -> Bus Creator/11  "R1Y"
  R1X/1 -> Bus Creator/10  "R1X"
  R2Y/1 -> Bus Creator/13  "R2Y"
  R2X/1 -> Bus Creator/12  "R2X"

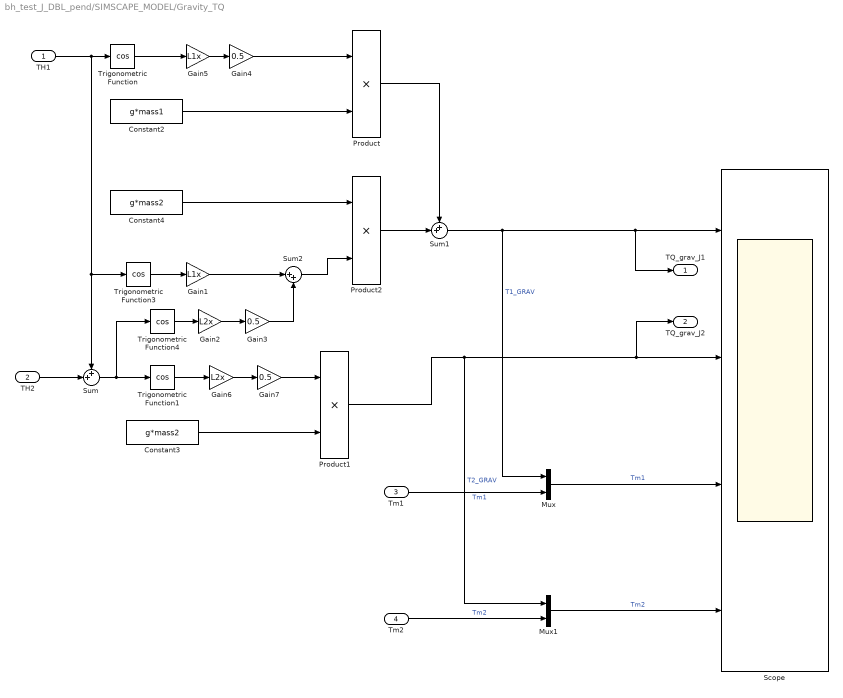
== system bh_test_J_DBL_pend/SIMSCAPE_MODEL/Gravity_TQ ==
  TH1 : Inport
  TH2 : Inport  Port=2
  Tm1 : Inport  Port=3
  Tm2 : Inport  Port=4
  Constant2 : Constant  Value=g*mass1
  Constant3 : Constant  Value=g*mass2
  Constant4 : Constant  Value=g*mass2
  Gain1 : Gain  Gain=L1x
  Gain2 : Gain  Gain=L2x
  Gain3 : Gain  Gain=0.5
  Gain4 : Gain  Gain=0.5
  Gain5 : Gain  Gain=L1x
  Gain6 : Gain  Gain=L2x
  Gain7 : Gain  Gain=0.5
  Mux : Mux  Inputs=2
  Mux1 : Mux  Inputs=2
  Product : Product
  Product1 : Product
  Product2 : Product
  Scope : Scope  NumInputPorts=4
  Sum : Sum  Inputs=++|
  Sum1 : Sum  Inputs=++|
  Sum2 : Sum  Inputs=|++
  Trigonometric Function{,1,3..4} (4 alike) : Trigonometry  Operator=cos
  TQ_grav_J1 : Outport
  TQ_grav_J2 : Outport  Port=2
  wires:
  TH2/1 -> Sum/2
  Sum/1 -> Trigonometric Function4/1, Trigonometric Function1/1
  Trigonometric Function/1 -> Gain5/1
  Trigonometric Function1/1 -> Gain6/1
  Constant3/1 -> Product1/2
  Product/1 -> Sum1/1
  TH1/1 -> Trigonometric Function/1, Trigonometric Function3/1, Sum/1
  Constant2/1 -> Product/2
  Constant4/1 -> Product2/1
  Trigonometric Function3/1 -> Gain1/1
  Gain1/1 -> Sum2/1
  Trigonometric Function4/1 -> Gain2/1
  Gain2/1 -> Gain3/1
  Gain3/1 -> Sum2/2
  Sum2/1 -> Product2/2
  Product2/1 -> Sum1/2
  Sum1/1 -> Mux/1, TQ_grav_J1/1, Scope/1  "T1_GRAV"
  Product1/1 -> Mux1/1, TQ_grav_J2/1, Scope/2  "T2_GRAV"
  Mux/1 -> Scope/3  "Tm1"
  Mux1/1 -> Scope/4  "Tm2"
  Tm1/1 -> Mux/2  "Tm1"
  Tm2/1 -> Mux1/2  "Tm2"
  Gain5/1 -> Gain4/1
  Gain4/1 -> Product/1
  Gain6/1 -> Gain7/1
  Gain7/1 -> Product1/1

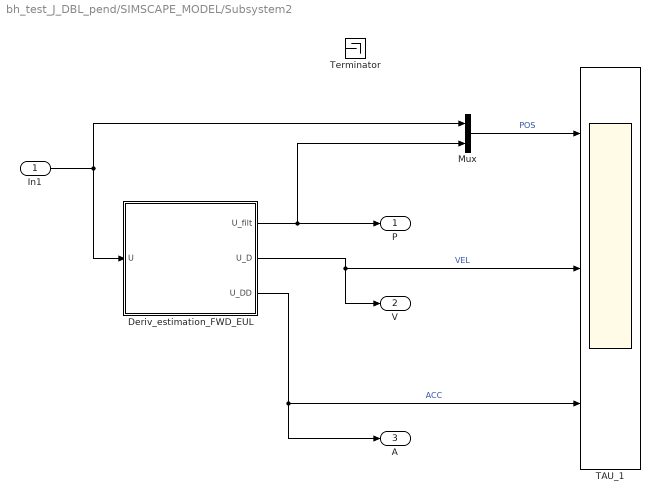
== system bh_test_J_DBL_pend/SIMSCAPE_MODEL/Subsystem2 ==
  In1 : Inport
  Deriv_estimation_FWD_EUL : Subsystem  mask(Derivative Estimation){wn=2*pi*25, p=1, dt=dt}
      mask prompts: wn "Natural frequency, wn (rad/sec)"; p "Damping ratio, p"; dt "Sample time, dt (secs)"
      mask help: A simple derivative estimator using a 2nd order representation between input and output.
      mask init:
      | str1 = sprintf('wn = %.2f', wn);
      | str2 = sprintf('p  = %.2f', p);
      | str3 = sprintf('dt = %.2f', dt);
      | str = char(str1,str2,str3);
      mask Display: disp(str)
  Mux : Mux  Inputs=2
  TAU_1 : Scope  NumInputPorts=3
  Terminator : Terminator
  P : Outport
  V : Outport  Port=2
  A : Outport  Port=3
  wires:
  In1/1 -> Deriv_estimation_FWD_EUL/1(U), Mux/1
  Deriv_estimation_FWD_EUL/1(U_filt) -> Mux/2, P/1
  Deriv_estimation_FWD_EUL/2(U_D) -> TAU_1/2, V/1  "VEL"
  Deriv_estimation_FWD_EUL/3(U_DD) -> TAU_1/3, A/1  "ACC"
  Mux/1 -> TAU_1/1  "POS"

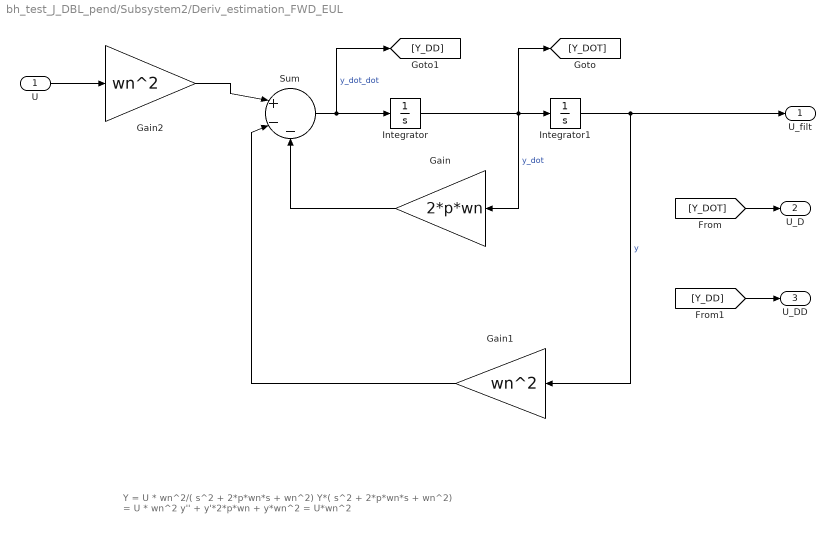
== system bh_test_J_DBL_pend/Subsystem2/Deriv_estimation_FWD_EUL ==
  note: Y = U *     wn^2/( s^2 + 2*p*wn*s + wn^2)
      | Y*( s^2 + 2*p*wn*s + wn^2) = U * wn^2
      |
      | y'' + y'*2*p*wn + y*wn^2 = U*wn^2
  U : Inport
  Gain : Gain  Gain=2*p*wn
  Gain1 : Gain  Gain=wn^2
  Gain2 : Gain  Gain=wn^2
  Integrator : Integrator
  Integrator1 : Integrator
  Sum : Sum  Inputs=|+--
  U_filt : Outport
  U_D : Outport  Port=2
  U_DD : Outport  Port=3
  wires:
  Integrator/1 -> Integrator1/1, [Y_DOT], Gain/1  "y_dot"
  Sum/1 -> [Y_DD], Integrator/1  "y_dot_dot"
  Integrator1/1 -> Gain1/1, U_filt/1  "y"
  U/1 -> Gain2/1
  Gain2/1 -> Sum/1
  Gain/1 -> Sum/3
  Gain1/1 -> Sum/2
  [Y_DOT] -> U_D/1
  [Y_DD] -> U_DD/1

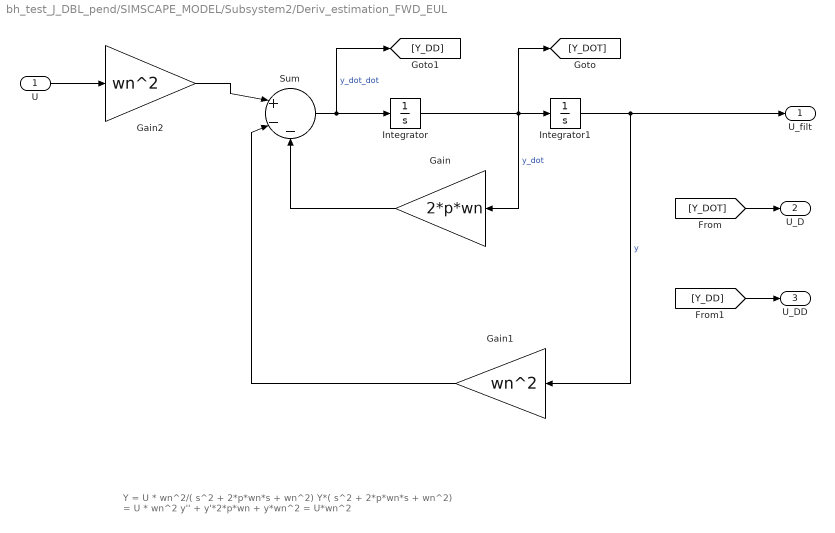
== system bh_test_J_DBL_pend/SIMSCAPE_MODEL/Subsystem2/Deriv_estimation_FWD_EUL ==
  note: Y = U *     wn^2/( s^2 + 2*p*wn*s + wn^2)
      | Y*( s^2 + 2*p*wn*s + wn^2) = U * wn^2
      |
      | y'' + y'*2*p*wn + y*wn^2 = U*wn^2
  U : Inport
  Gain : Gain  Gain=2*p*wn
  Gain1 : Gain  Gain=wn^2
  Gain2 : Gain  Gain=wn^2
  Integrator : Integrator
  Integrator1 : Integrator
  Sum : Sum  Inputs=|+--
  U_filt : Outport
  U_D : Outport  Port=2
  U_DD : Outport  Port=3
  wires:
  Integrator/1 -> Integrator1/1, [Y_DOT], Gain/1  "y_dot"
  Sum/1 -> [Y_DD], Integrator/1  "y_dot_dot"
  Integrator1/1 -> Gain1/1, U_filt/1  "y"
  U/1 -> Gain2/1
  Gain2/1 -> Sum/1
  Gain/1 -> Sum/3
  Gain1/1 -> Sum/2
  [Y_DOT] -> U_D/1
  [Y_DD] -> U_DD/1

== matlab function bh_test_J_DBL_pend/THE_XE_YE ==
  data: L_1 input; XE output; L_2 input; theta_1 input; theta_2 input; YE output
function [XE,YE] = THE_XEYE(L_1,L_2,theta_1,theta_2)
%#codegen

%    This function was generated by the Symbolic Math Toolbox version 7.0.
%    05-Sep-2016 11:23:53

XE = L_2.*cos(theta_1+theta_2)+L_1.*cos(theta_1);
if nargout > 1
    YE = L_2.*sin(theta_1+theta_2)+L_1.*sin(theta_1);
end

== matlab function bh_test_J_DBL_pend/THE_J ==
  data: L_1 input; the_J output; L_2 input; theta_1 input; theta_2 input
function the_J = THE_J(L_1,L_2,theta_1,theta_2)
%#codegen

%    This function was generated by the Symbolic Math Toolbox version 7.0.
%    05-Sep-2016 11:04:30

the_J = reshape([-L_2.*sin(theta_1+theta_2)-L_1.*sin(theta_1),L_2.*cos(theta_1+theta_2)+L_1.*cos(theta_1),-L_2.*sin(theta_1+theta_2),L_2.*cos(theta_1+theta_2)],[2,2]);

== matlab function bh_test_J_DBL_pend/MATLAB Function ==
  data: J input; the_cond output
function the_cond = COND(J)
%#codegen

the_cond = cond(J);

end

== matlab function bh_test_J_DBL_pend/CALC_THETA_DOT ==
  data: J input; TH_DOT output; XY_DOT input; lambda_sq input; alt_TH_DOT output
function [TH_DOT, alt_TH_DOT] = calc_TH_DOT(J, XY_DOT, lambda_sq)
%#codegen

    %% so our problem is this:
    %     J*q_dot = x_dot
    %
    % so a solution is:
    %
    %      q_dot = pinv(J) * x_dot
    
    TH_DOT = pinv(J) * XY_DOT;

    %% we can also penalise the q_dot by applying a weight to it.
    %  this will give us a solution where we get a "smaller" q_dot.  This
    %  acts as a "dampening" agent ... and we notice it most at startup.
    
    % consider solving the REGULARISED problem
    %     [       J_mxn  ] * q_dot =  [ x_dot ]
    %     [lamb^2*I_nxn  ]            [ 0_nx1 ]
    %
    % which we'll wite as:
    %
    %              new_A * q_dot = new_b
    %
    % so a solution is:
    %
    %      q_dot = pinv(new_A) * new_b
    
    [m, n]     = size(J); 
    I_mat      = eye( n ); 
    new_A      = [ J;
                   lambda_sq * I_mat];

    new_b      = [ XY_DOT;
                   zeros(n,1) ];

    alt_TH_DOT = pinv( new_A  ) * new_b;
end
